simulink model "lab5"  (R2021b)
settings: Solver=ode45  StartTime=0.0  StopTime=500  MaxStep=0.2  RelTol=1e-3  EnableMultiTasking=on
values from neighbouring files (symbols this model uses):
  ddMax = 3    [sysdata.m]
  deltaMax = 30    [sysdata.m]
  fConst = 0    [sysdata.m]
  K = 0.08    [lab2_otay.m]    (also in sysdata.m)
  Kc = 0.825    [sysdata.m]
  phiZad = 90    [sysdata.m]
  TI = 200    [sysdata.m]
  Toc = 5    [lab2_otay.m]    (also in sysdata.m)
  TR = 1    [lab2_otay.m]    (also in sysdata.m)
  Ts = 18.0    (= 18)    [lab2_otay.m]    (also in sysdata.m)
  Ts0 = Ts    [lab5go1.m]    (also in lab5go2.m)
settings Model: Creator=user  LastModifiedBy=Lapte
settings SolverCC: AlgebraicLoopSolver=TrustRegion
settings DataIOCC: LimitDataPoints=on  SaveFormat=Array  ReturnWorkspaceOutputs=off
settings OptimizationCC: LifeSpan=inf
settings DebuggingCC: SFUnexpectedBacktrackingDiag=warning  SFNoUnconditionalDefaultTransitionDiag=warning  SFExecutionAtInitializationDiag=none  SFMachineParentedDataDiag=warning  ArithmeticOperatorsInVariantConditions=warning
settings HardwareCC: ProdBitPerPointer=32  ProdBitPerSizeT=32  ProdBitPerPtrDiffT=32  ProdLargestAtomicFloat=None  ProdIntDivRoundTo=Undefined  ProdEndianess=Unspecified  ProdWordSize=32  ProdHWDeviceType=32-bit Generic
settings ModelReferenceCC: PropagateSignalLabelsOutOfModel=off
settings SFSimCC: SimUseLocalCustomCode=off  CustomCodeUndefinedFunction=UseInterfaceOnly
settings RTWCC: RTWUseLocalCustomCode=off
settings CodeAppCC: StateflowObjectComments=on
settings GRTTargetCC: TargetLangStandard=C89/C90 (ANSI)
settings ConfigComp: CovMetricSettings=dw  CovSaveCumulativeToWorkspaceVar=on  CovSaveSingleToWorkspaceVar=on  CovExternalEMLEnable=off  CovSFcnEnable=off

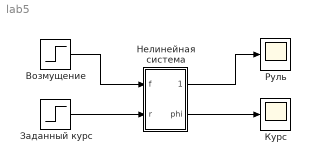
== system lab5 ==
  Возмущение : Step  Time=0  After=fConst  SampleTime=0
  Заданный курс : Step  Time=0  After=phiZad  SampleTime=0
  Курс : Scope
  Нелинейная система : Subsystem
  Руль : Scope
  wires:
  Возмущение/1 -> Нелинейная система/1(f)
  Заданный курс/1 -> Нелинейная система/2(r)
  Нелинейная система/1(delta) -> Руль/1
  Нелинейная система/2(phi) -> Курс/1

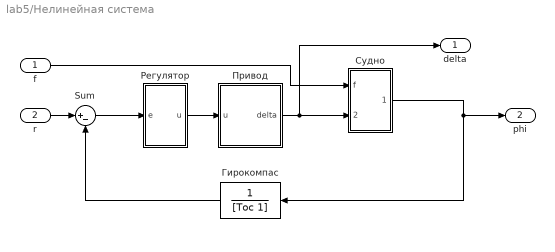
== system lab5/Нелинейная система ==
  f : Inport
  r : Inport  Port=2
  Sum : Sum  Inputs=|+-
  Гирокомпас : TransferFcn  Denominator=[Toc 1]
  Привод : Subsystem
  Регулятор : Subsystem
  Судно : Subsystem
  delta : Outport
  phi : Outport  Port=2
  wires:
  f/1 -> Судно/1(f)
  r/1 -> Sum/1
  Привод/1(delta) -> Судно/2(delta), delta/1
  Sum/1 -> Регулятор/1(e)
  Гирокомпас/1 -> Sum/2
  Судно/1(phi) -> Гирокомпас/1, phi/1
  Регулятор/1(u) -> Привод/1(u)

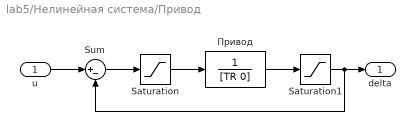
== system lab5/Нелинейная система/Привод ==
  u : Inport
  Saturation : Saturate  UpperLimit=TR*ddMax  LowerLimit=-TR*ddMax
  Saturation1 : Saturate  UpperLimit=deltaMax  LowerLimit=-deltaMax
  Sum : Sum  Inputs=|+-
  Привод : TransferFcn  Denominator=[TR 0]
  delta : Outport
  wires:
  Sum/1 -> Saturation/1
  u/1 -> Sum/1
  Saturation/1 -> Привод/1
  Привод/1 -> Saturation1/1
  Saturation1/1 -> delta/1, Sum/2

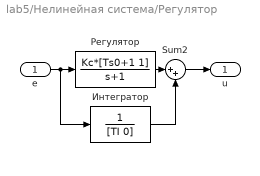
== system lab5/Нелинейная система/Регулятор ==
  e : Inport
  Sum2 : Sum  Inputs=|++
  Интегратор : TransferFcn  Denominator=[TI 0]
  Регулятор : TransferFcn  Numerator=Kc*[Ts0+1 1]  Denominator=[1 1]
  u : Outport
  wires:
  Sum2/1 -> u/1
  Регулятор/1 -> Sum2/1
  e/1 -> Регулятор/1, Интегратор/1
  Интегратор/1 -> Sum2/2

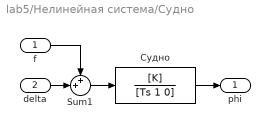
== system lab5/Нелинейная система/Судно ==
  f : Inport
  delta : Inport  Port=2
  Sum1 : Sum  Inputs=++|
  Судно : TransferFcn  Numerator=[K]  Denominator=[Ts 1 0]
  phi : Outport
  wires:
  Судно/1 -> phi/1
  f/1 -> Sum1/1
  Sum1/1 -> Судно/1
  delta/1 -> Sum1/2
